simulink model "Demo_PreScanCarSim3D_cs"  (Simulink 7.6)
settings: Solver=ode5  SolverMode=SingleTasking  StartTime=0.0  StopTime=68  FixedStep=1/400  RelTol=1e-3
model workspace (MAT data in the model file):
  mbox_table : struct (value not decoded)
PreLoadFcn:
  | check_NUTS_defined;
  | 
  | assignin('base',['model_closed_' bdroot],false);
InitFcn:
  | PreScanExperimentInitFcn(bdroot)
StopFcn:
  | PreScanExperimentStopFcn(bdroot)
undefined symbols (not defined in the file or in its folder): DiscIntNeverNeededParam, warningInitialVelocity, x0, x_ini_VRML, y_ini_VRML, z_ini_VRML
libraries: PreScanSimulinkLibrary x13, simulink_extras x5, PreScanUsefulBlocks x5, simulink x3, Solver_SF x1
(part 1 of 10)
CloseFcn:
  | evalin('base',['clear model_closed_' bdroot]);
settings Model: Creator=PRESCAN  LastModifiedBy=buildbot
settings OptimizationCC: BooleanDataType=off  InitFltsAndDblsToZero=on
settings DebuggingCC: SaveWithParameterizedLinksMsg=none  SignalResolutionControl=TryResolveAllWithWarning  SolverPrmCheckMsg=none  MultiTaskDSMMsg=warning  MultiTaskCondExecSysMsg=none
settings RTWCC: IncludeERTFirstTime=on
settings GRTTargetCC: TargetFcnLib=ansi_tfl_tmw.mat

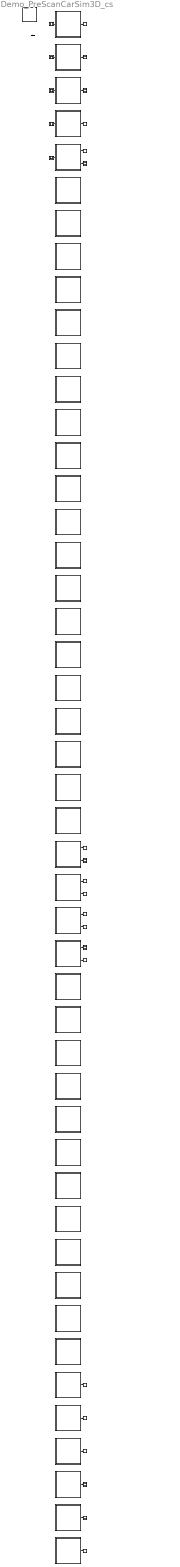
== system Demo_PreScanCarSim3D_cs ==
  note: Demo Help
  note: 7.1.4
  note: Regenerate
  note: Record for Replay
  note: Open Useful Blocks
  note: PreScan Options
  note: Version:
  note: 7.2.0
  note: Author(s):
  note: A. Pastore
  note: Descriptive text:
  note: PreScan CarSim-VehicleDynamics
      | coupling demo.
      | Actor used Audi A8.
  note: ID
      |
      | 952
      | 1033
      | 1034
      | 1035
      | 296
      | 639
      | 751
      | 761
      | 762
      | 763
      | 764
      | 765
      | 766
      | 767
      | 768
      | 769
      | 770
      | 771
      | 772
      | 773
      | 774
      | 775
      | 776
      | 777
      | 778
      | 115
      | 973
      | 985
      | 993
      | 456
      | 457
      | 458
      | 459
      | 460
      | 461
      | 462
      | 463
      | 464
      | 465
      | 560
      | 561
      | 499
      | 641
      | 642
      | 644
      | 645
      | 646
      | 647
      | 908
      | 909
      | 910
      | 911
      | 928
      | 929
      | 930
      | 931
  note: OBU-Beacon ID
  note: TypeID
      |
      | 5
      | 5
      | 5
      | 5
      | 1
      | 15
      | 15
      | 15
      | 15
      | 15
      | 15
      | 15
      | 15
      | 15
      | 15
      | 15
      | 15
      | 15
      | 15
      | 15
      | 15
      | 15
      | 15
      | 15
      | 15
      | 15
      | 15
      | 15
      | 15
      | 15
      | 15
      | 15
      | 15
      | 15
      | 15
      | 15
      | 15
      | 15
      | 15
      | 15
      | 15
      | 15
      | 15
      | 15
      | 15
      | 15
      | 15
      | 15
      | 15
      | 15
      | 15
      | 15
      | 15
      | 15
      | 15
      | 15
  note: TypeTag
      |
      | Cal element
      | Cal element
      | Cal element
      | Cal element
      | Car
      | Anim traffic sign
      | Anim traffic sign
      | Anim traffic sign
      | Anim traffic sign
      | Anim traffic sign
      | Anim traffic sign
      | Anim traffic sign
      | Anim traffic sign
      | Anim traffic sign
      | Anim traffic sign
      | Anim traffic sign
      | Anim traffic sign
      | Anim traffic sign
      | Anim traffic sign
      | Anim traffic sign
      | Anim traffic sign
      | Anim traffic sign
      | Anim traffic sign
      | Anim traffic sign
      | Anim traffic sign
      | Anim traffic sign
      | Anim traffic sign
      | Anim traffic sign
      | Anim traffic sign
      | Anim traffic sign
      | Anim traffic sign
      | Anim traffic sign
      | Anim traffic sign
      | Anim traffic sign
      | Anim traffic sign
      | Anim traffic sign
      | Anim traffic sign
      | Anim traffic sign
      | Anim traffic sign
      | Anim traffic sign
      | Anim traffic sign
      | Anim traffic sign
      | Anim traffic sign
      | Anim traffic sign
      | Anim traffic sign
      | Anim traffic sign
      | Anim traffic sign
      | Anim traffic sign
      | Anim traffic sign
      | Anim traffic sign
      | Anim traffic sign
      | Anim traffic sign
      | Anim traffic sign
      | Anim traffic sign
      | Anim traffic sign
      | Anim traffic sign
  note: SD
      |
      | Y
      | Y
      | Y
      | Y
      | Y
      | N
      | N
      | N
      | N
      | N
      | N
      | N
      | N
      | N
      | N
      | N
      | N
      | N
      | N
      | N
      | N
      | N
      | N
      | N
      | N
      | Y
      | Y
      | Y
      | Y
      | N
      | N
      | N
      | N
      | N
      | N
      | N
      | N
      | N
      | N
      | N
      | N
      | Y
      | Y
      | Y
      | Y
      | Y
      | Y
      | Y
      | Y
      | Y
      | Y
      | Y
      | Y
      | Y
      | Y
      | Y
  note: CD
      |
      | N
      | N
      | N
      | N
      | N
      | N
      | N
      | N
      | N
      | N
      | N
      | N
      | N
      | N
      | N
      | N
      | N
      | N
      | N
      | N
      | N
      | N
      | N
      | N
      | N
      | N
      | N
      | N
      | N
      | N
      | N
      | N
      | N
      | N
      | N
      | N
      | N
      | N
      | N
      | N
      | N
      | N
      | N
      | N
      | N
      | N
      | N
      | N
      | N
      | N
      | N
      | N
      | N
      | N
      | N
      | N
  note: Name
      |
      | Box_1
      | Box_2
      | Box_3
      | Box_4
      | Audi_A8_1
      | Lightpost_1
      | Lightpost_2
      | Lightpost_7
      | Lightpost_8
      | Lightpost_9
      | Lightpost_10
      | Lightpost_11
      | Lightpost_12
      | Lightpost_13
      | Lightpost_14
      | Lightpost_15
      | Lightpost_16
      | Lightpost_17
      | Lightpost_18
      | Lightpost_19
      | Lightpost_20
      | Lightpost_21
      | Lightpost_22
      | Lightpost_23
      | Lightpost_24
      | HighwayOverhang_1
      | HighwayOverhang_2
      | HighwayOverhang_3
      | HighwayOverhang_5
      | Lightpost_25
      | Lightpost_26
      | Lightpost_27
      | Lightpost_28
      | Lightpost_29
      | Lightpost_30
      | Lightpost_31
      | Lightpost_32
      | Lightpost_33
      | Lightpost_34
      | Lightpost_35
      | Lightpost_36
      | TrafficLightRoadSideNL_1
      | TrafficLightRoadSideNL_2
      | TrafficLightRoadSideNL_3
      | TrafficLightRoadSideNL_5
      | TrafficLightRoadSideNL_6
      | TrafficLightRoadSideNL_7
      | InformationBoard_2
      | InformationBoard_5
      | InformationBoard_6
      | InformationBoard_7
      | InformationBoard_8
      | InformationBoard_25
      | InformationBoard_26
      | InformationBoard_27
      | InformationBoard_28
  note: 7.4.0
  note: Num ID OBU-Beacon ID Type ID Type Tag SD CD Name
  Actuators : DataStoreMemory  Tag=Actuators  DataStoreName=SimCoreActuators  InitialValue=zeros(1236,1)
      settings: DeleteFcn=PreScanBlockDeleteFcn;
  Audi_A8_1 : Subsystem  Tag=WorldObjectSubSystem  InitFcn=UniqueId = '3037';
      mask Display: image(imread('Audi_A8.jpg'));color('white');text(0,0,' ID=296\n')
  Box_1 : Subsystem  Tag=WorldObjectSubSystem  InitFcn=UniqueId = '2076';
      mask Display: image(imread('Box.jpg'));color('white');text(0,0,' ID=952\n')
  Box_2 : Subsystem  Tag=WorldObjectSubSystem  InitFcn=UniqueId = '2077';
      mask Display: image(imread('Box.jpg'));color('white');text(0,0,' ID=1033\n')
  Box_3 : Subsystem  Tag=WorldObjectSubSystem  InitFcn=UniqueId = '2078';
      mask Display: image(imread('Box.jpg'));color('white');text(0,0,' ID=1034\n')
  Box_4 : Subsystem  Tag=WorldObjectSubSystem  InitFcn=UniqueId = '2079';
      mask Display: image(imread('Box.jpg'));color('white');text(0,0,' ID=1035\n')
  GetSensors : Subsystem  Tag=GetSensors  Priority=2  mask(PreScan Simulation Core Block){NrOfSensors=40, TimeStep=20/400}
      mask prompts: NrOfSensors "Number of sensor values"; TimeStep "Timestep [s]"
      mask help:
      | Please do not remove this block from the PreScan compilation sheet,
      | as it contains essential configuration parameters for a PreScan simulation.
      settings: DeleteFcn=PreScanBlockDeleteFcn;
  HighwayOverhang_1 : Subsystem  Tag=WorldObjectSubSystem  InitFcn=UniqueId = '1876';
      mask Display: image(imread('HighwayOverhang.jpg'));color('white');text(0,0,' ID=115\n')
  HighwayOverhang_2 : Subsystem  Tag=WorldObjectSubSystem  InitFcn=UniqueId = '1877';
      mask Display: image(imread('HighwayOverhang.jpg'));color('white');text(0,0,' ID=973\n')
  HighwayOverhang_3 : Subsystem  Tag=WorldObjectSubSystem  InitFcn=UniqueId = '1890';
      mask Display: image(imread('HighwayOverhang.jpg'));color('white');text(0,0,' ID=985\n')
  HighwayOverhang_5 : Subsystem  Tag=WorldObjectSubSystem  InitFcn=UniqueId = '1909';
      mask Display: image(imread('HighwayOverhang.jpg'));color('white');text(0,0,' ID=993\n')
  Lightpost_1 : Subsystem  Tag=WorldObjectSubSystem  InitFcn=UniqueId = '1495';
      mask Display: image(imread('Lightpost.jpg'));color('white');text(0,0,' ID=639\n')
  Lightpost_10 : Subsystem  Tag=WorldObjectSubSystem  InitFcn=UniqueId = '1504';
      mask Display: image(imread('Lightpost.jpg'));color('white');text(0,0,' ID=764\n')
  Lightpost_11 : Subsystem  Tag=WorldObjectSubSystem  InitFcn=UniqueId = '1505';
      mask Display: image(imread('Lightpost.jpg'));color('white');text(0,0,' ID=765\n')
  Lightpost_12 : Subsystem  Tag=WorldObjectSubSystem  InitFcn=UniqueId = '1506';
      mask Display: image(imread('Lightpost.jpg'));color('white');text(0,0,' ID=766\n')
  Lightpost_13 : Subsystem  Tag=WorldObjectSubSystem  InitFcn=UniqueId = '1507';
      mask Display: image(imread('Lightpost.jpg'));color('white');text(0,0,' ID=767\n')
  Lightpost_14 : Subsystem  Tag=WorldObjectSubSystem  InitFcn=UniqueId = '1508';
      mask Display: image(imread('Lightpost.jpg'));color('white');text(0,0,' ID=768\n')
  Lightpost_15 : Subsystem  Tag=WorldObjectSubSystem  InitFcn=UniqueId = '1509';
      mask Display: image(imread('Lightpost.jpg'));color('white');text(0,0,' ID=769\n')
  Lightpost_16 : Subsystem  Tag=WorldObjectSubSystem  InitFcn=UniqueId = '1510';
      mask Display: image(imread('Lightpost.jpg'));color('white');text(0,0,' ID=770\n')
  Lightpost_17 : Subsystem  Tag=WorldObjectSubSystem  InitFcn=UniqueId = '1511';
      mask Display: image(imread('Lightpost.jpg'));color('white');text(0,0,' ID=771\n')
  Lightpost_18 : Subsystem  Tag=WorldObjectSubSystem  InitFcn=UniqueId = '1512';
      mask Display: image(imread('Lightpost.jpg'));color('white');text(0,0,' ID=772\n')
  Lightpost_19 : Subsystem  Tag=WorldObjectSubSystem  InitFcn=UniqueId = '1513';
      mask Display: image(imread('Lightpost.jpg'));color('white');text(0,0,' ID=773\n')
  Lightpost_2 : Subsystem  Tag=WorldObjectSubSystem  InitFcn=UniqueId = '1496';
      mask Display: image(imread('Lightpost.jpg'));color('white');text(0,0,' ID=751\n')
  Lightpost_20 : Subsystem  Tag=WorldObjectSubSystem  InitFcn=UniqueId = '1514';
      mask Display: image(imread('Lightpost.jpg'));color('white');text(0,0,' ID=774\n')
  Lightpost_21 : Subsystem  Tag=WorldObjectSubSystem  InitFcn=UniqueId = '1515';
      mask Display: image(imread('Lightpost.jpg'));color('white');text(0,0,' ID=775\n')
  Lightpost_22 : Subsystem  Tag=WorldObjectSubSystem  InitFcn=UniqueId = '1516';
      mask Display: image(imread('Lightpost.jpg'));color('white');text(0,0,' ID=776\n')
  Lightpost_23 : Subsystem  Tag=WorldObjectSubSystem  InitFcn=UniqueId = '1517';
      mask Display: image(imread('Lightpost.jpg'));color('white');text(0,0,' ID=777\n')
  Lightpost_24 : Subsystem  Tag=WorldObjectSubSystem  InitFcn=UniqueId = '1518';
      mask Display: image(imread('Lightpost.jpg'));color('white');text(0,0,' ID=778\n')
  Lightpost_25 : Subsystem  Tag=WorldObjectSubSystem  InitFcn=UniqueId = '2334';
      mask Display: image(imread('Lightpost.jpg'));color('white');text(0,0,' ID=456\n')
  Lightpost_26 : Subsystem  Tag=WorldObjectSubSystem  InitFcn=UniqueId = '2335';
      mask Display: image(imread('Lightpost.jpg'));color('white');text(0,0,' ID=457\n')
  Lightpost_27 : Subsystem  Tag=WorldObjectSubSystem  InitFcn=UniqueId = '2336';
      mask Display: image(imread('Lightpost.jpg'));color('white');text(0,0,' ID=458\n')
  Lightpost_28 : Subsystem  Tag=WorldObjectSubSystem  InitFcn=UniqueId = '2337';
      mask Display: image(imread('Lightpost.jpg'));color('white');text(0,0,' ID=459\n')
  Lightpost_29 : Subsystem  Tag=WorldObjectSubSystem  InitFcn=UniqueId = '2338';
      mask Display: image(imread('Lightpost.jpg'));color('white');text(0,0,' ID=460\n')
  Lightpost_30 : Subsystem  Tag=WorldObjectSubSystem  InitFcn=UniqueId = '2339';
      mask Display: image(imread('Lightpost.jpg'));color('white');text(0,0,' ID=461\n')
  Lightpost_31 : Subsystem  Tag=WorldObjectSubSystem  InitFcn=UniqueId = '2340';
      mask Display: image(imread('Lightpost.jpg'));color('white');text(0,0,' ID=462\n')
  Lightpost_32 : Subsystem  Tag=WorldObjectSubSystem  InitFcn=UniqueId = '2341';
      mask Display: image(imread('Lightpost.jpg'));color('white');text(0,0,' ID=463\n')
  Lightpost_33 : Subsystem  Tag=WorldObjectSubSystem  InitFcn=UniqueId = '2342';
      mask Display: image(imread('Lightpost.jpg'));color('white');text(0,0,' ID=464\n')
  Lightpost_34 : Subsystem  Tag=WorldObjectSubSystem  InitFcn=UniqueId = '2343';
      mask Display: image(imread('Lightpost.jpg'));color('white');text(0,0,' ID=465\n')
  Lightpost_35 : Subsystem  Tag=WorldObjectSubSystem  InitFcn=UniqueId = '2473';
      mask Display: image(imread('Lightpost.jpg'));color('white');text(0,0,' ID=560\n')
  Lightpost_36 : Subsystem  Tag=WorldObjectSubSystem  InitFcn=UniqueId = '2474';
      mask Display: image(imread('Lightpost.jpg'));color('white');text(0,0,' ID=561\n')
  Lightpost_7 : Subsystem  Tag=WorldObjectSubSystem  InitFcn=UniqueId = '1501';
      mask Display: image(imread('Lightpost.jpg'));color('white');text(0,0,' ID=761\n')
  Lightpost_8 : Subsystem  Tag=WorldObjectSubSystem  InitFcn=UniqueId = '1502';
      mask Display: image(imread('Lightpost.jpg'));color('white');text(0,0,' ID=762\n')
  Lightpost_9 : Subsystem  Tag=WorldObjectSubSystem  InitFcn=UniqueId = '1503';
      mask Display: image(imread('Lightpost.jpg'));color('white');text(0,0,' ID=763\n')
  SELF_Audi_A8_1 : Subsystem  Tag=SELF  Priority=3  mask(PreScan Source Block: SELF){PortName=SELF_Audi_A8_1, PortIndex=32, PortWidth=8, TimeStep=20/400}
      mask prompts: PortName "Auto-Assigned: Port Name [-]"; PortIndex "Auto-Assigned: Port Index [-]"; PortWidth "Auto-Assigned: Port Dimensions"; TimeStep "Auto-Assigned: Upload Period [s]"
      mask help:
      | The SELF port shows (state) information of the actor itself. The outputs are position in the experiment's axis system and the GPS coordinates, and the object's absolute velocity and compass heading.
      |
      | For more information, please click Help.
      settings: DeleteFcn=PreScanBlockDeleteFcn;
      mask Help: eval('openHelp(462)')
      mask Display: image(imread('GPS.png'))
  SELF_Box_1 : Subsystem  Tag=SELF  Priority=3  mask(PreScan Source Block: SELF){PortName=SELF_Box_1, PortIndex=0, PortWidth=8, TimeStep=20/400}
      mask prompts: PortName "Auto-Assigned: Port Name [-]"; PortIndex "Auto-Assigned: Port Index [-]"; PortWidth "Auto-Assigned: Port Dimensions"; TimeStep "Auto-Assigned: Upload Period [s]"
      mask help:
      | The SELF port shows (state) information of the actor itself. The outputs are position in the experiment's axis system and the GPS coordinates, and the object's absolute velocity and compass heading.
      |
      | For more information, please click Help.
      settings: DeleteFcn=PreScanBlockDeleteFcn;
      mask Help: eval('openHelp(462)')
      mask Display: image(imread('GPS.png'))
  SELF_Box_2 : Subsystem  Tag=SELF  Priority=3  mask(PreScan Source Block: SELF){PortName=SELF_Box_2, PortIndex=8, PortWidth=8, TimeStep=20/400}
      mask prompts: PortName "Auto-Assigned: Port Name [-]"; PortIndex "Auto-Assigned: Port Index [-]"; PortWidth "Auto-Assigned: Port Dimensions"; TimeStep "Auto-Assigned: Upload Period [s]"
      mask help:
      | The SELF port shows (state) information of the actor itself. The outputs are position in the experiment's axis system and the GPS coordinates, and the object's absolute velocity and compass heading.
      |
      | For more information, please click Help.
      settings: DeleteFcn=PreScanBlockDeleteFcn;
      mask Help: eval('openHelp(462)')
      mask Display: image(imread('GPS.png'))
  SELF_Box_3 : Subsystem  Tag=SELF  Priority=3  mask(PreScan Source Block: SELF){PortName=SELF_Box_3, PortIndex=16, PortWidth=8, TimeStep=20/400}
      mask prompts: PortName "Auto-Assigned: Port Name [-]"; PortIndex "Auto-Assigned: Port Index [-]"; PortWidth "Auto-Assigned: Port Dimensions"; TimeStep "Auto-Assigned: Upload Period [s]"
      mask help:
      | The SELF port shows (state) information of the actor itself. The outputs are position in the experiment's axis system and the GPS coordinates, and the object's absolute velocity and compass heading.
      |
      | For more information, please click Help.
      settings: DeleteFcn=PreScanBlockDeleteFcn;
      mask Help: eval('openHelp(462)')
      mask Display: image(imread('GPS.png'))
  SELF_Box_4 : Subsystem  Tag=SELF  Priority=3  mask(PreScan Source Block: SELF){PortName=SELF_Box_4, PortIndex=24, PortWidth=8, TimeStep=20/400}
      mask prompts: PortName "Auto-Assigned: Port Name [-]"; PortIndex "Auto-Assigned: Port Index [-]"; PortWidth "Auto-Assigned: Port Dimensions"; TimeStep "Auto-Assigned: Upload Period [s]"
      mask help:
      | The SELF port shows (state) information of the actor itself. The outputs are position in the experiment's axis system and the GPS coordinates, and the object's absolute velocity and compass heading.
      |
      | For more information, please click Help.
      settings: DeleteFcn=PreScanBlockDeleteFcn;
      mask Help: eval('openHelp(462)')
      mask Display: image(imread('GPS.png'))
  STATE_Audi_A8_1 : Subsystem  Tag=State  Priority=0  mask(PreScan Sink Block: State){x0=-21.039824129566149, y0=-15.143190800389089, z0=0.241, Roll0=0, Pitch0=0, Yaw0=0.029771632590382069, TimeStep=20/400}
      mask prompts: x0 "Ini x-position VEHICLE wrt GLOBAL axis system [m]"; y0 "Ini y-position VEHICLE wrt GLOBAL axis system [m]"; z0 "Ini z-position VEHICLE wrt GLOBAL axis system [m]"; Roll0 "Ini roll-angle BODY wrt VEHICLE axis system [deg]"; Pitch0 "Ini pitch-angle BODY wrt VEHICLE axis system [deg]"; Yaw0 "Ini yaw-angle VEHICLE wrt GLOBAL axis system [deg]"; TimeStep "Time Step [s]"
      mask help:
      | The Actor State contains a vector signal of size (9x1), containing the following signals:
      |
      | -  Position                  (x,y,z)                                     [m]
      | -  Velocity                  (vx,vy,vz)                               [m/s]
      | -  Angles                    (Roll, Pitch, Yaw)                   [rad]
      |
      | The Actor state is defined in the global axis system.
      | The state is superponed on the Initial position defined in the GUI.
      |
      | For more information, please click Help.
      settings: DeleteFcn=PreScanBlockDeleteFcn;
      mask Help: eval('openHelp(222)')
      mask Display: image(imread('State.png'))
  STATE_Box_1 : Subsystem  Tag=State  Priority=0  mask(PreScan Sink Block: State){x0=340, y0=0, z0=2.45, Roll0=0, Pitch0=0, Yaw0=0, TimeStep=20/400}
      mask prompts: x0 "Ini x-position VEHICLE wrt GLOBAL axis system [m]"; y0 "Ini y-position VEHICLE wrt GLOBAL axis system [m]"; z0 "Ini z-position VEHICLE wrt GLOBAL axis system [m]"; Roll0 "Ini roll-angle BODY wrt VEHICLE axis system [deg]"; Pitch0 "Ini pitch-angle BODY wrt VEHICLE axis system [deg]"; Yaw0 "Ini yaw-angle VEHICLE wrt GLOBAL axis system [deg]"; TimeStep "Time Step [s]"
      mask help:
      | The Actor State contains a vector signal of size (9x1), containing the following signals:
      |
      | -  Position                  (x,y,z)                                     [m]
      | -  Velocity                  (vx,vy,vz)                               [m/s]
      | -  Angles                    (Roll, Pitch, Yaw)                   [rad]
      |
      | The Actor state is defined in the global axis system.
      | The state is superponed on the Initial position defined in the GUI.
      |
      | For more information, please click Help.
      settings: DeleteFcn=PreScanBlockDeleteFcn;
      mask Help: eval('openHelp(222)')
      mask Display: image(imread('State.png'))
  STATE_Box_2 : Subsystem  Tag=State  Priority=0  mask(PreScan Sink Block: State){x0=345, y0=0, z0=2.45, Roll0=0, Pitch0=0, Yaw0=0, TimeStep=20/400}
      mask prompts: x0 "Ini x-position VEHICLE wrt GLOBAL axis system [m]"; y0 "Ini y-position VEHICLE wrt GLOBAL axis system [m]"; z0 "Ini z-position VEHICLE wrt GLOBAL axis system [m]"; Roll0 "Ini roll-angle BODY wrt VEHICLE axis system [deg]"; Pitch0 "Ini pitch-angle BODY wrt VEHICLE axis system [deg]"; Yaw0 "Ini yaw-angle VEHICLE wrt GLOBAL axis system [deg]"; TimeStep "Time Step [s]"
      mask help:
      | The Actor State contains a vector signal of size (9x1), containing the following signals:
      |
      | -  Position                  (x,y,z)                                     [m]
      | -  Velocity                  (vx,vy,vz)                               [m/s]
      | -  Angles                    (Roll, Pitch, Yaw)                   [rad]
      |
      | The Actor state is defined in the global axis system.
      | The state is superponed on the Initial position defined in the GUI.
      |
      | For more information, please click Help.
      settings: DeleteFcn=PreScanBlockDeleteFcn;
      mask Help: eval('openHelp(222)')
      mask Display: image(imread('State.png'))
  STATE_Box_3 : Subsystem  Tag=State  Priority=0  mask(PreScan Sink Block: State){x0=350, y0=0, z0=2.45, Roll0=0, Pitch0=0, Yaw0=0, TimeStep=20/400}
      mask prompts: x0 "Ini x-position VEHICLE wrt GLOBAL axis system [m]"; y0 "Ini y-position VEHICLE wrt GLOBAL axis system [m]"; z0 "Ini z-position VEHICLE wrt GLOBAL axis system [m]"; Roll0 "Ini roll-angle BODY wrt VEHICLE axis system [deg]"; Pitch0 "Ini pitch-angle BODY wrt VEHICLE axis system [deg]"; Yaw0 "Ini yaw-angle VEHICLE wrt GLOBAL axis system [deg]"; TimeStep "Time Step [s]"
      mask help:
      | The Actor State contains a vector signal of size (9x1), containing the following signals:
      |
      | -  Position                  (x,y,z)                                     [m]
      | -  Velocity                  (vx,vy,vz)                               [m/s]
      | -  Angles                    (Roll, Pitch, Yaw)                   [rad]
      |
      | The Actor state is defined in the global axis system.
      | The state is superponed on the Initial position defined in the GUI.
      |
      | For more information, please click Help.
      settings: DeleteFcn=PreScanBlockDeleteFcn;
      mask Help: eval('openHelp(222)')
      mask Display: image(imread('State.png'))
  STATE_Box_4 : Subsystem  Tag=State  Priority=0  mask(PreScan Sink Block: State){x0=345, y0=0, z0=4.55, Roll0=0, Pitch0=0, Yaw0=0, TimeStep=20/400}
      mask prompts: x0 "Ini x-position VEHICLE wrt GLOBAL axis system [m]"; y0 "Ini y-position VEHICLE wrt GLOBAL axis system [m]"; z0 "Ini z-position VEHICLE wrt GLOBAL axis system [m]"; Roll0 "Ini roll-angle BODY wrt VEHICLE axis system [deg]"; Pitch0 "Ini pitch-angle BODY wrt VEHICLE axis system [deg]"; Yaw0 "Ini yaw-angle VEHICLE wrt GLOBAL axis system [deg]"; TimeStep "Time Step [s]"
      mask help:
      | The Actor State contains a vector signal of size (9x1), containing the following signals:
      |
      | -  Position                  (x,y,z)                                     [m]
      | -  Velocity                  (vx,vy,vz)                               [m/s]
      | -  Angles                    (Roll, Pitch, Yaw)                   [rad]
      |
      | The Actor state is defined in the global axis system.
      | The state is superponed on the Initial position defined in the GUI.
      |
      | For more information, please click Help.
      settings: DeleteFcn=PreScanBlockDeleteFcn;
      mask Help: eval('openHelp(222)')
      mask Display: image(imread('State.png'))
  SetActuators : Subsystem  Tag=SetActuators  Priority=1  mask(PreScan Simulation Core Block){TimeStep=20/400, NrOfActuators=1236}
      mask prompts: TimeStep "Timestep [s]"; NrOfActuators "Number of actuator values"
      mask help:
      | Please do not remove this block from the PreScan compilation sheet,
      | as it contains essential configuration parameters for a PreScan simulation.
      settings: DeleteFcn=PreScanBlockDeleteFcn;
  SimCoreConfiguration : M-S-Function  Tag=SimCoreConfiguration  Description=0737A9264C5EAA56F51D361F6C986A2357CB2C6EC5B4C73B5560DE9525D1CE72  FunctionName=SimCoreBlock  Parameters=ExperimentXML PortsXML SimulationCore HostName CheckStart EnableLog RfR EnableGPUAccel ShowComputationTime  mask(PreScan Simulation Core Configurator){SimulationCore=NUTS, HostName=0, CheckStart=0, prescanversion='7.4.0', EnableLog=off, RfR=0, EnableGPUAccel=off, ShowComputationTime=off}
      mask prompts: SimulationCore "Simulation Core"; HostName "Simulation Host"; CheckStart "Show START Dialog"; prescanversion "PreScan Version"; EnableLog "Create TA Log"; RfR "Record for Replay"; EnableGPUAccel "Enable GPU Acceleration"; ShowComputationTime "Show ComputationTime Scope"
      mask help:
      | Please do not remove this block from the PreScan compilation sheet,
      | as it contains essential configuration parameter for a PreScan simulation.
      mask init:
      | model = bdroot;
      | ExperimentXML = [model(1:end-3) '.pex'];
      | PortsXML = [model '_ports.pcd'];
      settings: DeleteFcn=PreScanBlockDeleteFcn;  ModelCloseFcn=assignin('base',['model_closed_' bdroot],true);  PreSaveFcn=disableSIDWarnings();  PostSaveFcn=enableSIDWarnings();
      mask Help: eval('openHelp(812)')
      mask Display: image(imread('prescanlogo.ico'))
  SimCoreInfo : Subsystem  Tag=SimCoreInfo
  TrafficLightRoadSideNL_1 : Subsystem  Tag=WorldObjectSubSystem  InitFcn=UniqueId = '2553';
      mask Display: image(imread('TrafficLightRoadSideNL.jpg'));color('white');text(0,0,' ID=499\n')
  TrafficLightRoadSideNL_2 : Subsystem  Tag=WorldObjectSubSystem  InitFcn=UniqueId = '2554';
      mask Display: image(imread('TrafficLightRoadSideNL.jpg'));color('white');text(0,0,' ID=641\n')
  TrafficLightRoadSideNL_3 : Subsystem  Tag=WorldObjectSubSystem  InitFcn=UniqueId = '2555';
      mask Display: image(imread('TrafficLightRoadSideNL.jpg'));color('white');text(0,0,' ID=642\n')
  TrafficLightRoadSideNL_5 : Subsystem  Tag=WorldObjectSubSystem  InitFcn=UniqueId = '2557';
      mask Display: image(imread('TrafficLightRoadSideNL.jpg'));color('white');text(0,0,' ID=644\n')
  TrafficLightRoadSideNL_6 : Subsystem  Tag=WorldObjectSubSystem  InitFcn=UniqueId = '2558';
      mask Display: image(imread('TrafficLightRoadSideNL.jpg'));color('white');text(0,0,' ID=645\n')
  TrafficLightRoadSideNL_7 : Subsystem  Tag=WorldObjectSubSystem  InitFcn=UniqueId = '2559';
      mask Display: image(imread('TrafficLightRoadSideNL.jpg'));color('white');text(0,0,' ID=646\n')
  VISUCasingLights_TrafficLightRoadSideNL_1 : Subsystem  Tag=VisuCasingLights  Priority=0
      settings: DeleteFcn=PreScanBlockDeleteFcn;
      mask Type: PreScan Sink Block: VisuLights
      mask Description:
      | The VisuLights block provides a way to animate the indicator and braking lights of a vehicle.
      | 
      | For more information, please click Help.
      mask Help: eval('openHelp(223)')
      mask Display: image(imread('TrafficLightCasing.png'))
  VISUCasingLights_TrafficLightRoadSideNL_2 : Subsystem  Tag=VisuCasingLights  Priority=0
      settings: DeleteFcn=PreScanBlockDeleteFcn;
      mask Type: PreScan Sink Block: VisuLights
      mask Description:
      | The VisuLights block provides a way to animate the indicator and braking lights of a vehicle.
      | 
      | For more information, please click Help.
      mask Help: eval('openHelp(223)')
      mask Display: image(imread('TrafficLightCasing.png'))
  VISUCasingLights_TrafficLightRoadSideNL_3 : Subsystem  Tag=VisuCasingLights  Priority=0
      settings: DeleteFcn=PreScanBlockDeleteFcn;
      mask Type: PreScan Sink Block: VisuLights
      mask Description:
      | The VisuLights block provides a way to animate the indicator and braking lights of a vehicle.
      | 
      | For more information, please click Help.
      mask Help: eval('openHelp(223)')
      mask Display: image(imread('TrafficLightCasing.png'))
  VISUCasingLights_TrafficLightRoadSideNL_5 : Subsystem  Tag=VisuCasingLights  Priority=0
      settings: DeleteFcn=PreScanBlockDeleteFcn;
      mask Type: PreScan Sink Block: VisuLights
      mask Description:
      | The VisuLights block provides a way to animate the indicator and braking lights of a vehicle.
      | 
      | For more information, please click Help.
      mask Help: eval('openHelp(223)')
      mask Display: image(imread('TrafficLightCasing.png'))
  VISUCasingLights_TrafficLightRoadSideNL_6 : Subsystem  Tag=VisuCasingLights  Priority=0
      settings: DeleteFcn=PreScanBlockDeleteFcn;
      mask Type: PreScan Sink Block: VisuLights
      mask Description:
      | The VisuLights block provides a way to animate the indicator and braking lights of a vehicle.
      | 
      | For more information, please click Help.
      mask Help: eval('openHelp(223)')
      mask Display: image(imread('TrafficLightCasing.png'))
  VISUCasingLights_TrafficLightRoadSideNL_7 : Subsystem  Tag=VisuCasingLights  Priority=0
      settings: DeleteFcn=PreScanBlockDeleteFcn;
      mask Type: PreScan Sink Block: VisuLights
      mask Description:
      | The VisuLights block provides a way to animate the indicator and braking lights of a vehicle.
      | 
      | For more information, please click Help.
      mask Help: eval('openHelp(223)')
      mask Display: image(imread('TrafficLightCasing.png'))
  VISUMatrixSignLights_HighwayOverhang_1 : Subsystem  Tag=VisuMatrixSignLights  Priority=0
      settings: DeleteFcn=PreScanBlockDeleteFcn;
      mask Type: PreScan Sink Block: VisuMatrixSign
      mask Description:
      | The VisuMatrixSign block provides a way to adapt the texture of the plates connected to an overhang, based on Resource IDs of the texture files.
      | 
      | For more information, please click Help.
      mask Help: eval('openHelp()')
      mask Display: image(imread('HighwaySpeedMatrix.png'))
  VISUMatrixSignLights_HighwayOverhang_2 : Subsystem  Tag=VisuMatrixSignLights  Priority=0
      settings: DeleteFcn=PreScanBlockDeleteFcn;
      mask Type: PreScan Sink Block: VisuMatrixSign
      mask Description:
      | The VisuMatrixSign block provides a way to adapt the texture of the plates connected to an overhang, based on Resource IDs of the texture files.
      | 
      | For more information, please click Help.
      mask Help: eval('openHelp()')
      mask Display: image(imread('HighwaySpeedMatrix.png'))
  VISUMatrixSignLights_HighwayOverhang_3 : Subsystem  Tag=VisuMatrixSignLights  Priority=0
      settings: DeleteFcn=PreScanBlockDeleteFcn;
      mask Type: PreScan Sink Block: VisuMatrixSign
      mask Description:
      | The VisuMatrixSign block provides a way to adapt the texture of the plates connected to an overhang, based on Resource IDs of the texture files.
      | 
      | For more information, please click Help.
      mask Help: eval('openHelp()')
      mask Display: image(imread('HighwaySpeedMatrix.png'))
  VISUMatrixSignLights_HighwayOverhang_5 : Subsystem  Tag=VisuMatrixSignLights  Priority=0
      settings: DeleteFcn=PreScanBlockDeleteFcn;
      mask Type: PreScan Sink Block: VisuMatrixSign
      mask Description:
      | The VisuMatrixSign block provides a way to adapt the texture of the plates connected to an overhang, based on Resource IDs of the texture files.
      | 
      | For more information, please click Help.
      mask Help: eval('openHelp()')
      mask Display: image(imread('HighwaySpeedMatrix.png'))
  VISUMatrixSign_HighwayOverhang_1 : Subsystem  Tag=VisuMatrixSign  Priority=0
      settings: DeleteFcn=PreScanBlockDeleteFcn;
      mask Type: PreScan Sink Block: VisuMatrixSign
      mask Description:
      | The VisuMatrixSign block provides a way to adapt the texture of the plates connected to an overhang, based on Resource IDs of the texture files.
      | 
      | For more information, please click Help.
      mask Help: eval('openHelp()')
      mask Display: image(imread('HighwaySpeedMatrix.png'))
  VISUMatrixSign_HighwayOverhang_2 : Subsystem  Tag=VisuMatrixSign  Priority=0
      settings: DeleteFcn=PreScanBlockDeleteFcn;
      mask Type: PreScan Sink Block: VisuMatrixSign
      mask Description:
      | The VisuMatrixSign block provides a way to adapt the texture of the plates connected to an overhang, based on Resource IDs of the texture files.
      | 
      | For more information, please click Help.
      mask Help: eval('openHelp()')
      mask Display: image(imread('HighwaySpeedMatrix.png'))
  VISUMatrixSign_HighwayOverhang_3 : Subsystem  Tag=VisuMatrixSign  Priority=0
      settings: DeleteFcn=PreScanBlockDeleteFcn;
      mask Type: PreScan Sink Block: VisuMatrixSign
      mask Description:
      | The VisuMatrixSign block provides a way to adapt the texture of the plates connected to an overhang, based on Resource IDs of the texture files.
      | 
      | For more information, please click Help.
      mask Help: eval('openHelp()')
      mask Display: image(imread('HighwaySpeedMatrix.png'))
  VISUMatrixSign_HighwayOverhang_5 : Subsystem  Tag=VisuMatrixSign  Priority=0
      settings: DeleteFcn=PreScanBlockDeleteFcn;
      mask Type: PreScan Sink Block: VisuMatrixSign
      mask Description:
      | The VisuMatrixSign block provides a way to adapt the texture of the plates connected to an overhang, based on Resource IDs of the texture files.
      | 
      | For more information, please click Help.
      mask Help: eval('openHelp()')
      mask Display: image(imread('HighwaySpeedMatrix.png'))
  VISUWheelsCarSim_Audi_A8_1 : Subsystem  Tag=VisuWheels  Priority=0
      settings: DeleteFcn=PreScanBlockDeleteFcn;
      mask Type: PreScan Sink Block: VisuWheels
      mask Description:
      | The VisuWheels block provides a way to animate the wheels of a vehicle, with steering, rotation (because of velocity) and z-displacement.
      | 
      | For more information, please click Help.
      mask Help: eval('openHelp(223)')
      mask Display: image(imread('wheel.png'))
  wires:
  SetActuators/1(dummy) -> GetSensors/1(dummy)
  TrafficLightRoadSideNL_7/1(VISUCasingLights_TrafficLightRoadSideNL_7) -> VISUCasingLights_TrafficLightRoadSideNL_7/1(CasingLights)
  TrafficLightRoadSideNL_6/1(VISUCasingLights_TrafficLightRoadSideNL_6) -> VISUCasingLights_TrafficLightRoadSideNL_6/1(CasingLights)
  TrafficLightRoadSideNL_5/1(VISUCasingLights_TrafficLightRoadSideNL_5) -> VISUCasingLights_TrafficLightRoadSideNL_5/1(CasingLights)
  TrafficLightRoadSideNL_3/1(VISUCasingLights_TrafficLightRoadSideNL_3) -> VISUCasingLights_TrafficLightRoadSideNL_3/1(CasingLights)
  TrafficLightRoadSideNL_2/1(VISUCasingLights_TrafficLightRoadSideNL_2) -> VISUCasingLights_TrafficLightRoadSideNL_2/1(CasingLights)
  TrafficLightRoadSideNL_1/1(VISUCasingLights_TrafficLightRoadSideNL_1) -> VISUCasingLights_TrafficLightRoadSideNL_1/1(CasingLights)
  HighwayOverhang_5/2(VISUMatrixSignLights_HighwayOverhang_5) -> VISUMatrixSignLights_HighwayOverhang_5/1(MatrixSignLights)
  HighwayOverhang_5/1(VISUMatrixSign_HighwayOverhang_5) -> VISUMatrixSign_HighwayOverhang_5/1(MatrixSigns)
  HighwayOverhang_3/2(VISUMatrixSignLights_HighwayOverhang_3) -> VISUMatrixSignLights_HighwayOverhang_3/1(MatrixSignLights)
  HighwayOverhang_3/1(VISUMatrixSign_HighwayOverhang_3) -> VISUMatrixSign_HighwayOverhang_3/1(MatrixSigns)
  HighwayOverhang_2/2(VISUMatrixSignLights_HighwayOverhang_2) -> VISUMatrixSignLights_HighwayOverhang_2/1(MatrixSignLights)
  HighwayOverhang_2/1(VISUMatrixSign_HighwayOverhang_2) -> VISUMatrixSign_HighwayOverhang_2/1(MatrixSigns)
  HighwayOverhang_1/2(VISUMatrixSignLights_HighwayOverhang_1) -> VISUMatrixSignLights_HighwayOverhang_1/1(MatrixSignLights)
  HighwayOverhang_1/1(VISUMatrixSign_HighwayOverhang_1) -> VISUMatrixSign_HighwayOverhang_1/1(MatrixSigns)
  Audi_A8_1/2(VISUWheelsCarSim_Audi_A8_1) -> VISUWheelsCarSim_Audi_A8_1/1(Wheels)
  SELF_Audi_A8_1/1(U) -> Audi_A8_1/1(SELF_Audi_A8_1)
  Audi_A8_1/1(STATE_Audi_A8_1) -> STATE_Audi_A8_1/1(State)
  SELF_Box_4/1(U) -> Box_4/1(SELF_Box_4)
  Box_4/1(STATE_Box_4) -> STATE_Box_4/1(State)
  SELF_Box_3/1(U) -> Box_3/1(SELF_Box_3)
  Box_3/1(STATE_Box_3) -> STATE_Box_3/1(State)
  SELF_Box_2/1(U) -> Box_2/1(SELF_Box_2)
  Box_2/1(STATE_Box_2) -> STATE_Box_2/1(State)
  SELF_Box_1/1(U) -> Box_1/1(SELF_Box_1)
  Box_1/1(STATE_Box_1) -> STATE_Box_1/1(State)

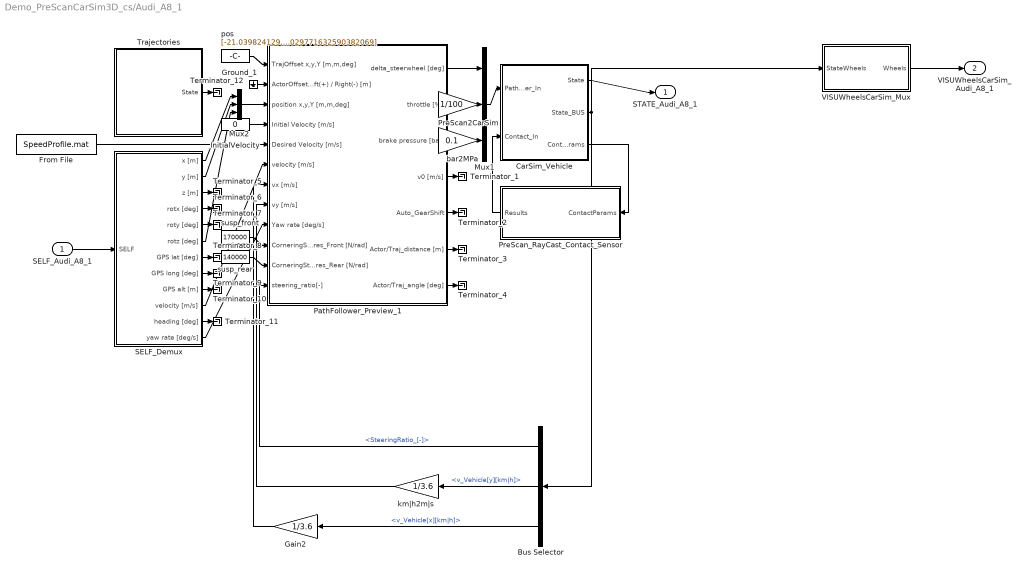
== system Demo_PreScanCarSim3D_cs/Audi_A8_1 ==
  SELF_Audi_A8_1 : Inport  Tag=SELFInport
  Bus Selector : BusSelector  OutputSignals=PreScanBUS_VehicleDynamics.Steering.SteeringRatio_[-],PreScanBUS_VehicleDynamics.Vehicle.Velocities.Linear.v_Vehicle[y][km|h],PreScanBUS_VehicleDynamics.Vehicle.Velocities.Linear.v_Vehicle[x][km|h]
  CarSim_Vehicle : Subsystem  Tag=UserSpecified_Subsys  Description=.\CarSim_Data\Extensions\Simulink\CarSim_VehicleDynamics.mdl  mask(User specified subsystem){update=off, sourcefilename=.\\CarSim_Data\\Extensions\\Simulink\\CarSim_VehicleDynamics.mdl}
      mask prompts: update "Update (default: not checked)"; sourcefilename "Source file name"
      mask help:
      | A User-specified model may be selected as Controller or Dynamics of the vehicle. PreScan will copy the contents of the User-specified model into the user-specified model block.
      |
      | If update checkbox is checked the current user-specified model block will be deleted and will be REPLACED by (new) user specified model blocks. So, the current user specified model elements will be lost.
      |
      | Warning: If a new user-specified model is selected in the GUI, the user-specified model will be replaced.
      settings: DeleteFcn=PreScanBlockDeleteFcn;
      mask Help: eval('openHelp(227)')
      mask Display: image(imread('UserSpecDyn.png')); port_label('output', 1, 'State'); port_label('output', 2, 'State_Bus'); port_label('output', 3, 'ContactParams'); text(0,0,' CarSim Vehicle\n')
  From File : FromFile  FileName=SpeedProfile.mat  SampleTime=eval(get_param(bdroot,'FixedStep'))
  Gain2 : Gain  Gain=1/3.6
  Ground_1 : Ground
  InitialVelocity : Constant  Tag=InitialVelocity  Value=0
  Mux1 : Mux  Inputs=3
  Mux2 : Mux  Inputs=3
  PathFollower_Preview_1 : Subsystem  Tag=PathFollower_Preview  mask(PreScan Block: Path Follower with Preview){Migrate=on, FileName='Trajectory_1.mat', mass=1820, Jzz=4095, length_a=1.265, length_l=2.947, Angle_Max_SteeringWheel=500, PreviewTime=0.8, DelayTime=0.1, LowSpeedLimit=20, MaxSteeringRate=1200, CSSampleTime=1/400, PFIntegrationFrequency=100}
      mask prompts: Migrate "Migrate. During migration this block will be replaced by a newer one."; FileName "Trajectory Name"; mass "Mass vehicle total [kg]"; Jzz "Inertia vehicle around yaw axis [kg m2]"; length_a "Distance between COG and front axle [m]"; length_l "Length of wheelbase [m]"; Angle_Max_SteeringWheel "Maximum steering wheel angle [deg]"; PreviewTime "Preview time [s]"; DelayTime "Delay time [s]"; LowSpeedLimit "Low-speed limit [km/h]"; MaxSteeringRate "Maximum steering wheel angle rate [deg/s]"; CSSampleTime "Compilation Sheet sample time [s]"; PFIntegrationFrequency "Lateral controller frequency [Hz]"
      mask help:
      | The Path Follower Model is selected in the GUI to simulate driver behavior.
      |
      | For more information, please click Help.
      mask init:
      | load(['trajectories/',eval(FileName)])
      | traject=trajectory';
      | 
      | Traj_x=traject(:,2);
      | Traj_y=traject(:,3);
      | Traj_t=traject(2,1);
      | Traj_v=sqrt(traject(:,8).^2+traject(:,9).^2+traject(:,10).^2);
      | 
      | RefreshCounter = (1/CSSampleTime) / (PFIntegrationFrequency); %Compilation sheet frequency/path follower frequency
      | 
      | blockPath = gcb;
      | 
      | clear traject;
      mask Help: eval('openHelp(233)')
  PreScan2CarSim : Gain  Gain=1/100
  PreScan_RayCast_Contact_Sensor : Subsystem  Tag=PreScan_RayCast_Contact_Sensor  mask(PreScan Block: PreScan RayCast Contact Sensor){x0=-21.039824129566149, y0=-15.143190800389089, z0=0.241, Roll0=0, Pitch0=0, Yaw0=0.029771632590382069, wheelRadius=0.358, hcog=0.241, b=2.947, TimeStep=-1}
      mask prompts: x0 "Ini x-position VEHICLE wrt GLOBAL axis system [m]"; y0 "Ini y-position VEHICLE wrt GLOBAL axis system [m]"; z0 "Ini z-position VEHICLE wrt GLOBAL axis system [m]"; Roll0 "Ini roll-angle BODY wrt VEHICLE axis system [deg]"; Pitch0 "Ini pitch-angle BODY wrt VEHICLE axis system [deg]"; Yaw0 "Ini yaw-angle VEHICLE wrt GLOBAL axis system [deg]"; wheelRadius "Wheel Radius [m]"; hcog "Dynamics: hCoG [m]"; b "Dynamics: b [m]"; TimeStep "Time Step [s]"
      mask help:
      | This block encapsulates the base Contact sensor.
      |
      | It takes input parameters from the PreScan 3D vehicle dynamics block and outputs contact results.
      mask Help: eval('openHelp(251)')
  SELF_Demux : Subsystem  Tag=DemuxSELF
      settings: DeleteFcn=PreScanBlockDeleteFcn;
      mask Type: PreScan Demux Block:
      mask Display:
      | port_label('output',1,'x [m]')
      | port_label('output',2,'y [m]')
      | port_label('output',3,'z [m]','texmode','on')
      | port_label('output',4,'Rotx [deg]','texmode','on')
      | port_label('output',5,'Roty [deg]','texmode','on')
      | port_label('output',6,'Rotz [deg]','texmode','on')
      | port_label('output',7,'GPS lat [deg]','texmode','on')
      | port_label('output',8,'GPS long [deg]','texmode','on')
      | port_label('output',9,'GPS alt [m]','texmode','on')
      | port_label('output',10,'Velocity [m/s]')
      | port_label('output',11,'Heading [deg]')
      | port_label('output',12,'Yaw rate [deg/s]')
  Terminator_{1..12} (12 alike) : Terminator
  Trajectories : Subsystem  Tag=Trajectories
      settings: DeleteFcn=PreScanBlockDeleteFcn;
      mask Type: PreScan Source Block: Trajectories
      mask Description:
      | The Trajectory block contains the trajectories defined in the PreScan Experiment Editor. The output of the trajectory block is the (vehicle) State.
      | 
      | For more information, please click Help.
      mask Help: eval('openHelp(312)')
      mask Display: image(imread('Trajectory.png'));
  VISUWheelsCarSim_Mux : Subsystem  Tag=MuxWheels  mask(PreScan Mux Block:){TimeStep=-1}
      mask prompts: TimeStep "Auto Assigned: Time Step [s]"
      settings: DeleteFcn=PreScanBlockDeleteFcn;
  bar2MPa : Gain  Gain=0.1
  km|h2m|s : Gain  Gain=1/3.6
  pos : Constant  Tag=pos  Value=[-21.039824129566149 -15.143190800389089 0.029771632590382069]
  susp_front : Constant  Tag=susp_front  Value=170000
  susp_rear : Constant  Tag=susp_rear  Value=140000
  STATE_Audi_A8_1 : Outport  Tag=StateOutport
  VISUWheelsCarSim_Audi_A8_1 : Outport  Tag=VisuWheelsOutport  Port=2  SampleTime=20/400
  wires:
  Bus Selector/2 -> km|h2m|s/1  "<v_Vehicle[y][km|h]>"
  Bus Selector/3 -> Gain2/1  "<v_Vehicle[x][km|h]>"
  PreScan2CarSim/1 -> Mux1/2
  bar2MPa/1 -> Mux1/3
  Trajectories/1(State) -> Terminator_12/1
  SELF_Demux/11(heading [deg]) -> Terminator_11/1
  SELF_Demux/9(GPS alt [m]) -> Terminator_10/1
  SELF_Demux/8(GPS long [deg]) -> Terminator_9/1
  SELF_Demux/7(GPS lat [deg]) -> Terminator_8/1
  SELF_Demux/5(roty [deg]) -> Terminator_7/1
  SELF_Demux/4(rotx [deg]) -> Terminator_6/1
  SELF_Demux/3(z [m]) -> Terminator_5/1
  PathFollower_Preview_1/7(Actor/Traj_angle [deg]) -> Terminator_4/1
  PathFollower_Preview_1/6(Actor/Traj_distance [m]) -> Terminator_3/1
  PathFollower_Preview_1/5(Auto_GearShift) -> Terminator_2/1
  PathFollower_Preview_1/4(v0 [m/s]) -> Terminator_1/1
  Ground_1/1 -> PathFollower_Preview_1/2(ActorOffset_Left(+) / Right(-) [m])
  CarSim_Vehicle/2(State_BUS) -> VISUWheelsCarSim_Mux/1(StateWheels), Bus Selector/1
  PathFollower_Preview_1/1(delta_steerwheel [deg]) -> Mux1/1
  SELF_Demux/1(x [m]) -> Mux2/1
  SELF_Demux/2(y [m]) -> Mux2/2
  SELF_Demux/6(rotz [deg]) -> Mux2/3
  Mux2/1 -> PathFollower_Preview_1/3(position x,y,Y [m,m,deg])
  Bus Selector/1 -> PathFollower_Preview_1/12(steering_ratio[-])  "<SteeringRatio_[-]>"
  km|h2m|s/1 -> PathFollower_Preview_1/8(vy [m/s])
  Gain2/1 -> PathFollower_Preview_1/7(vx [m/s])
  Mux1/1 -> CarSim_Vehicle/1(PathFollower_In)
  PathFollower_Preview_1/2(throttle [%]) -> PreScan2CarSim/1
  From File/1 -> PathFollower_Preview_1/5(Desired Velocity [m/s])
  PathFollower_Preview_1/3(brake pressure [bar]) -> bar2MPa/1
  SELF_Demux/10(velocity [m/s]) -> PathFollower_Preview_1/6(velocity [m/s])
  SELF_Demux/12(yaw rate [deg/s]) -> PathFollower_Preview_1/9(Yaw rate [deg/s])
  PreScan_RayCast_Contact_Sensor/1(Results) -> CarSim_Vehicle/2(Contact_In)
  CarSim_Vehicle/3(ContactParams) -> PreScan_RayCast_Contact_Sensor/1(ContactParams)
  CarSim_Vehicle/1(State) -> STATE_Audi_A8_1/1
  VISUWheelsCarSim_Mux/1(Wheels) -> VISUWheelsCarSim_Audi_A8_1/1
  SELF_Audi_A8_1/1 -> SELF_Demux/1(SELF)
  susp_rear/1 -> PathFollower_Preview_1/11(CorneringStiffness_Tyres_Rear [N/rad])
  susp_front/1 -> PathFollower_Preview_1/10(CorneringStiffness_Tyres_Front [N/rad])
  InitialVelocity/1 -> PathFollower_Preview_1/4(Initial Velocity [m/s])
  pos/1 -> PathFollower_Preview_1/1(TrajOffset x,y,Y [m,m,deg])

== system Demo_PreScanCarSim3D_cs/Box_1 ==
  SELF_Box_1 : Inport  Tag=SELFInport
  Dynamics_Empty : Subsystem  Tag=Dynamics_Empty
      mask Display: port_label('output', 1, 'State');text(0,0,' Empty\n')
  SELF_Demux : Subsystem  Tag=DemuxSELF
      settings: DeleteFcn=PreScanBlockDeleteFcn;
      mask Type: PreScan Demux Block:
      mask Display:
      | port_label('output',1,'x [m]')
      | port_label('output',2,'y [m]')
      | port_label('output',3,'z [m]','texmode','on')
      | port_label('output',4,'Rotx [deg]','texmode','on')
      | port_label('output',5,'Roty [deg]','texmode','on')
      | port_label('output',6,'Rotz [deg]','texmode','on')
      | port_label('output',7,'GPS lat [deg]','texmode','on')
      | port_label('output',8,'GPS long [deg]','texmode','on')
      | port_label('output',9,'GPS alt [m]','texmode','on')
      | port_label('output',10,'Velocity [m/s]')
      | port_label('output',11,'Heading [deg]')
      | port_label('output',12,'Yaw rate [deg/s]')
  Terminator_{1..12} (12 alike) : Terminator
  STATE_Box_1 : Outport  Tag=StateOutport
  wires:
  SELF_Demux/12(yaw rate [deg/s]) -> Terminator_12/1
  SELF_Demux/11(heading [deg]) -> Terminator_11/1
  SELF_Demux/10(velocity [m/s]) -> Terminator_10/1
  SELF_Demux/9(GPS alt [m]) -> Terminator_9/1
  SELF_Demux/8(GPS long [deg]) -> Terminator_8/1
  SELF_Demux/7(GPS lat [deg]) -> Terminator_7/1
  SELF_Demux/6(rotz [deg]) -> Terminator_6/1
  SELF_Demux/5(roty [deg]) -> Terminator_5/1
  SELF_Demux/4(rotx [deg]) -> Terminator_4/1
  SELF_Demux/3(z [m]) -> Terminator_3/1
  SELF_Demux/2(y [m]) -> Terminator_2/1
  SELF_Demux/1(x [m]) -> Terminator_1/1
  Dynamics_Empty/1(State) -> STATE_Box_1/1
  SELF_Box_1/1 -> SELF_Demux/1(SELF)

== system Demo_PreScanCarSim3D_cs/Box_2 ==
  SELF_Box_2 : Inport  Tag=SELFInport
  Dynamics_Empty : Subsystem  Tag=Dynamics_Empty
      mask Display: port_label('output', 1, 'State');text(0,0,' Empty\n')
  SELF_Demux : Subsystem  Tag=DemuxSELF
      settings: DeleteFcn=PreScanBlockDeleteFcn;
      mask Type: PreScan Demux Block:
      mask Display:
      | port_label('output',1,'x [m]')
      | port_label('output',2,'y [m]')
      | port_label('output',3,'z [m]','texmode','on')
      | port_label('output',4,'Rotx [deg]','texmode','on')
      | port_label('output',5,'Roty [deg]','texmode','on')
      | port_label('output',6,'Rotz [deg]','texmode','on')
      | port_label('output',7,'GPS lat [deg]','texmode','on')
      | port_label('output',8,'GPS long [deg]','texmode','on')
      | port_label('output',9,'GPS alt [m]','texmode','on')
      | port_label('output',10,'Velocity [m/s]')
      | port_label('output',11,'Heading [deg]')
      | port_label('output',12,'Yaw rate [deg/s]')
  Terminator_{1..12} (12 alike) : Terminator
  STATE_Box_2 : Outport  Tag=StateOutport
  wires:
  SELF_Demux/12(yaw rate [deg/s]) -> Terminator_12/1
  SELF_Demux/11(heading [deg]) -> Terminator_11/1
  SELF_Demux/10(velocity [m/s]) -> Terminator_10/1
  SELF_Demux/9(GPS alt [m]) -> Terminator_9/1
  SELF_Demux/8(GPS long [deg]) -> Terminator_8/1
  SELF_Demux/7(GPS lat [deg]) -> Terminator_7/1
  SELF_Demux/6(rotz [deg]) -> Terminator_6/1
  SELF_Demux/5(roty [deg]) -> Terminator_5/1
  SELF_Demux/4(rotx [deg]) -> Terminator_4/1
  SELF_Demux/3(z [m]) -> Terminator_3/1
  SELF_Demux/2(y [m]) -> Terminator_2/1
  SELF_Demux/1(x [m]) -> Terminator_1/1
  Dynamics_Empty/1(State) -> STATE_Box_2/1
  SELF_Box_2/1 -> SELF_Demux/1(SELF)

== system Demo_PreScanCarSim3D_cs/Box_3 ==
  SELF_Box_3 : Inport  Tag=SELFInport
  Dynamics_Empty : Subsystem  Tag=Dynamics_Empty
      mask Display: port_label('output', 1, 'State');text(0,0,' Empty\n')
  SELF_Demux : Subsystem  Tag=DemuxSELF
      settings: DeleteFcn=PreScanBlockDeleteFcn;
      mask Type: PreScan Demux Block:
      mask Display:
      | port_label('output',1,'x [m]')
      | port_label('output',2,'y [m]')
      | port_label('output',3,'z [m]','texmode','on')
      | port_label('output',4,'Rotx [deg]','texmode','on')
      | port_label('output',5,'Roty [deg]','texmode','on')
      | port_label('output',6,'Rotz [deg]','texmode','on')
      | port_label('output',7,'GPS lat [deg]','texmode','on')
      | port_label('output',8,'GPS long [deg]','texmode','on')
      | port_label('output',9,'GPS alt [m]','texmode','on')
      | port_label('output',10,'Velocity [m/s]')
      | port_label('output',11,'Heading [deg]')
      | port_label('output',12,'Yaw rate [deg/s]')
  Terminator_{1..12} (12 alike) : Terminator
  STATE_Box_3 : Outport  Tag=StateOutport
  wires:
  SELF_Demux/12(yaw rate [deg/s]) -> Terminator_12/1
  SELF_Demux/11(heading [deg]) -> Terminator_11/1
  SELF_Demux/10(velocity [m/s]) -> Terminator_10/1
  SELF_Demux/9(GPS alt [m]) -> Terminator_9/1
  SELF_Demux/8(GPS long [deg]) -> Terminator_8/1
  SELF_Demux/7(GPS lat [deg]) -> Terminator_7/1
  SELF_Demux/6(rotz [deg]) -> Terminator_6/1
  SELF_Demux/5(roty [deg]) -> Terminator_5/1
  SELF_Demux/4(rotx [deg]) -> Terminator_4/1
  SELF_Demux/3(z [m]) -> Terminator_3/1
  SELF_Demux/2(y [m]) -> Terminator_2/1
  SELF_Demux/1(x [m]) -> Terminator_1/1
  Dynamics_Empty/1(State) -> STATE_Box_3/1
  SELF_Box_3/1 -> SELF_Demux/1(SELF)

== system Demo_PreScanCarSim3D_cs/Box_4 ==
  SELF_Box_4 : Inport  Tag=SELFInport
  Dynamics_Empty : Subsystem  Tag=Dynamics_Empty
      mask Display: port_label('output', 1, 'State');text(0,0,' Empty\n')
  SELF_Demux : Subsystem  Tag=DemuxSELF
      settings: DeleteFcn=PreScanBlockDeleteFcn;
      mask Type: PreScan Demux Block:
      mask Display:
      | port_label('output',1,'x [m]')
      | port_label('output',2,'y [m]')
      | port_label('output',3,'z [m]','texmode','on')
      | port_label('output',4,'Rotx [deg]','texmode','on')
      | port_label('output',5,'Roty [deg]','texmode','on')
      | port_label('output',6,'Rotz [deg]','texmode','on')
      | port_label('output',7,'GPS lat [deg]','texmode','on')
      | port_label('output',8,'GPS long [deg]','texmode','on')
      | port_label('output',9,'GPS alt [m]','texmode','on')
      | port_label('output',10,'Velocity [m/s]')
      | port_label('output',11,'Heading [deg]')
      | port_label('output',12,'Yaw rate [deg/s]')
  Terminator_{1..12} (12 alike) : Terminator
  STATE_Box_4 : Outport  Tag=StateOutport
  wires:
  SELF_Demux/12(yaw rate [deg/s]) -> Terminator_12/1
  SELF_Demux/11(heading [deg]) -> Terminator_11/1
  SELF_Demux/10(velocity [m/s]) -> Terminator_10/1
  SELF_Demux/9(GPS alt [m]) -> Terminator_9/1
  SELF_Demux/8(GPS long [deg]) -> Terminator_8/1
  SELF_Demux/7(GPS lat [deg]) -> Terminator_7/1
  SELF_Demux/6(rotz [deg]) -> Terminator_6/1
  SELF_Demux/5(roty [deg]) -> Terminator_5/1
  SELF_Demux/4(rotx [deg]) -> Terminator_4/1
  SELF_Demux/3(z [m]) -> Terminator_3/1
  SELF_Demux/2(y [m]) -> Terminator_2/1
  SELF_Demux/1(x [m]) -> Terminator_1/1
  Dynamics_Empty/1(State) -> STATE_Box_4/1
  SELF_Box_4/1 -> SELF_Demux/1(SELF)
